simulink model "v2021_10_27_Modello_SITL_AENEA_2020b"  (R2020b)
settings: Solver=ode4  StartTime=0.0  StopTime=150  FixedStep=0.01  RelTol=1e-3
values from neighbouring files (symbols this model uses):
  alphavec_rad = [-0.10471975512 -0.0872664625997 -0.0698131700798 -0.0523598775598 -0.0349065850399 -0.0174532925199 0 0.0174532925199 0.0349065850399 0.0523598775598 0.0698131700798 0.0872664625997 ... (13 elements, 1x13)]    [datiAerodinamiciAENEA.mat]    (also in v2021_10_27_calcoloAerodinamica.m = deg2rad(alphavec))
  attuatore_Amax = 20*(pi/180)    (= 0.349065850399)    [v2021_10_27_avvioSITL.m]    (also in v2021_10_27_calcoloAerodinamica.m)
  attuatore_Emax = 25*(pi/180)    (= 0.436332312999)    [v2021_10_27_avvioSITL.m]    (also in v2021_10_27_calcoloAerodinamica.m)
  attuatore_Rmax = 25*(pi/180)    (= 0.436332312999)    [v2021_10_27_avvioSITL.m]    (also in v2021_10_27_calcoloAerodinamica.m)
  b = 2.62    [datiAerodinamiciAENEA.mat]    (also in derivateROSKAM_new.m; v2021_10_27_calcoloAerodinamica.m)
  beta_phi = 1/10.5600    (= 0.094696969697)    [Load_modello_sensori.m]
  beta_psi = 1/170    (= 0.00588235294118)    [Load_modello_sensori.m]
  beta_theta = 1/10.5000    (= 0.0952380952381)    [Load_modello_sensori.m]
  betavec_rad = [-0.209439510239 -0.13962634016 -0.0698131700798 0 0.0698131700798 0.13962634016 0.209439510239]    [datiAerodinamiciAENEA.mat]    (also in v2021_10_27_calcoloAerodinamica.m = deg2rad(betavec))
  c = 0.32    [datiAerodinamiciAENEA.mat]    (also in derivateROSKAM_new.m; v2021_10_27_calcoloAerodinamica.m)
  cbar = 0.32    [datiAerodinamiciAENEA.mat]    (also in v2021_10_27_calcoloAerodinamica.m)
  CD0 = 0.2    [datiAerodinamiciAENEA.mat]    (also in v2021_10_27_calcoloAerodinamica.m = 0.024)
  CldA = KCldA(1)*180/pi    [Alettoni.m]    (also in datiAerodinamiciAENEA.mat = 0.490103315517)
  CLdE = KCLdE(1)*180/pi    [Equilibratore.m]    (also in datiAerodinamiciAENEA.mat = 0.809101149087)
  CldR = 0.0568697125654    [datiAerodinamiciAENEA.mat]
  Clp = -0.4318    [datiAerodinamiciAENEA.mat]    (also in derivateROSKAM_new.m = clp_w+2*(Zv/b)^2*cy_betav+Clp_tail; v2021_10_27_calcoloAerodinamica.m)
  CLq = 8.13    [datiAerodinamiciAENEA.mat]    (also in v2021_10_27_calcoloAerodinamica.m)
  Clr = 0.1459    [datiAerodinamiciAENEA.mat]    (also in derivateROSKAM_new.m = cl*clr_cl-(2/b^2)*(lv*cos(alpha)+Zv*sin(alpha))*(Zv*cos(alph; v2021_10_27_calcoloAerodinamica.m)
  CmdE = KCmdE(1)*180/pi    [Equilibratore.m]    (also in datiAerodinamiciAENEA.mat = -3.59730623976)
  Cmq = -23.24    [datiAerodinamiciAENEA.mat]    (also in derivateROSKAM_new.m = -K*cL_alphaw*((AR*(2*(Xw/c)^2+0.5*(Xw/c))/(AR+2))+1/8)-2*cL_; v2021_10_27_calcoloAerodinamica.m)
  CndA = KCndA(1)*180/pi    [Alettoni.m]    (also in datiAerodinamiciAENEA.mat = -0.0456969018066)
  CndR = -0.162544523826    [datiAerodinamiciAENEA.mat]
  Cnp = 0.000294    [datiAerodinamiciAENEA.mat]    (also in derivateROSKAM_new.m = -clp_w*tan(alpha)+Clp*tan(alpha)-(2/b)*(lv*cos(alpha)+Zv*sin; v2021_10_27_calcoloAerodinamica.m = 0.007507)
  Cnr = -0.4872    [datiAerodinamiciAENEA.mat]    (also in derivateROSKAM_new.m = (Cnr_Clquadro)*cl^2+(cnr_cd0)*cd0+(2/b^2)*(lv*cos(alpha)+Zv*; v2021_10_27_calcoloAerodinamica.m)
  CYdA = KCYdA(1)*180/pi    [Alettoni.m]    (also in datiAerodinamiciAENEA.mat = -0.0146577407549)
  CYdR = -0.298131751664    [datiAerodinamiciAENEA.mat]
  CYp = 0.050728    [datiAerodinamiciAENEA.mat]    (also in v2021_10_27_calcoloAerodinamica.m)
  CYr = 0.358925    [datiAerodinamiciAENEA.mat]    (also in v2021_10_27_calcoloAerodinamica.m)
  delay_ahrs = 0    [Load_modello_sensori.m]
  delay_bmp = 0    [Load_modello_sensori.m]
  delay_gps = 0    [Load_modello_sensori.m]
  deltaAtrim = 0    [v2021_10_27_avvioSITL.m]
  deltaEtrim = (Cm0*CL_alpharad+Cm_alpharad*CLtrim)/(CL_alpharad*CmdE)    [calcoloDatiIniziali.m]    (also in v2021_10_27_avvioSITL.m = 0)
  deltaRtrim = 0    [v2021_10_27_avvioSITL.m]
  deltaTtrim = 0.1    [v2021_10_27_avvioSITL.m]
  Dprop = 0.5334    [datiAerodinamiciAENEA.mat]    (also in v2021_10_27_calcoloAerodinamica.m)
  g = [0 0 9.81]    [datiAerodinamiciAENEA.mat]    (also in v2021_10_27_calcoloAerodinamica.m = [0 0 9.81]')
  HINI = -State0.Pos0(3)    [v2021_10_27_avvioSITL.m]
  J_vec = [0 0.03 0.06 0.09 0.11 0.14 0.17 0.2 0.23 0.26 0.28 0.31 ... (30 elements, 30x1)]    [datiAerodinamiciAENEA.mat]
  Jeng = 0    [datiAerodinamiciAENEA.mat]    (also in v2021_10_27_calcoloAerodinamica.m)
  Jprop = 0.00422031414    [datiAerodinamiciAENEA.mat]    (also in v2021_10_27_calcoloAerodinamica.m)
  latitudineINI = 41.88754294247101*pi/180    (= 0.731075539917)    [v2021_10_27_avvioSITL.m]
  longitudineINI = 12.539364533818434*pi/180    (= 0.218853197223)    [v2021_10_27_avvioSITL.m]
  mean_ax = 0*0.0392    (= 0)    [Load_modello_sensori.m]
  mean_ay = -0*0.0598    (= 0)    [Load_modello_sensori.m]
  mean_az = 0*0.0384    (= 0)    [Load_modello_sensori.m]
  mean_p = 0*1.5184e-06    (= 0)    [Load_modello_sensori.m]
  mean_q = 0*2.9671e-05    (= 0)    [Load_modello_sensori.m]
  mean_r = 0*5.4105e-05    (= 0)    [Load_modello_sensori.m]
  P_ref = 1.0074e+05    (= 100740)    [Load_modello_sensori.m]
  PWM_Aileron = rad2deg(deltaAtrim)*9+1503    [v2021_10_27_avvioSITL.m]
  PWM_Elevator = rad2deg(deltaEtrim)*(447/50)+(3007/2)    [v2021_10_27_avvioSITL.m]
  PWM_Rudder = rad2deg(deltaRtrim)*(447/50)+(3007/2)    [v2021_10_27_avvioSITL.m]
  PWM_Throttle = (deltaTtrim)*800+1100    (= 1180)    [v2021_10_27_avvioSITL.m]
  q = prediction(11)    [f_pred_F1B.m]
  r = prediction(12)    [f_pred_F1B.m]
  rACtG = [-1.334 0 -0.2103]    [datiAerodinamiciAENEA.mat]    (also in v2021_10_27_calcoloAerodinamica.m = rACtP-rGP)
  rACwG = [-0.0589 0 -0.1645]    [datiAerodinamiciAENEA.mat]    (also in v2021_10_27_calcoloAerodinamica.m = rACwP-rGP)
  rAHRSG = [0 0 0.1075]    [datiAerodinamiciAENEA.mat]    (also in v2021_10_27_calcoloAerodinamica.m = rAHRSP-rGP)
  rho = 1.2133    [datiAerodinamiciAENEA.mat]    (also in derivateROSKAM_new.m = 1.16123787958; v2021_10_27_calcoloAerodinamica.m)
  rLEG = [0.0211 0 -0.1645]    [datiAerodinamiciAENEA.mat]    (also in v2021_10_27_calcoloAerodinamica.m = rLEP-rGP)
  rmglG = [-0.2319 -0.2 0.3925]    [datiAerodinamiciAENEA.mat]    (also in v2021_10_27_calcoloAerodinamica.m = rmglP-rGP)
  rmgrG = [-0.2319 0.2 0.3925]    [datiAerodinamiciAENEA.mat]    (also in v2021_10_27_calcoloAerodinamica.m = rmgrP-rGP)
  rngG = [0.2969 0 0.3925]    [datiAerodinamiciAENEA.mat]    (also in v2021_10_27_calcoloAerodinamica.m = rngP-rGP)
  rNPG = [-0.2442 0 -0.1645]    [datiAerodinamiciAENEA.mat]    (also in v2021_10_27_calcoloAerodinamica.m = rNPP-rGP)
  rPG = [0.5 0 -0.1075]    [datiAerodinamiciAENEA.mat]    (also in v2021_10_27_calcoloAerodinamica.m = -rGP)
  Rprop = 0.2667    [datiAerodinamiciAENEA.mat]    (also in v2021_10_27_calcoloAerodinamica.m)
  S = 0.8384    [datiAerodinamiciAENEA.mat]    (also in derivateROSKAM_new.m; v2021_10_27_calcoloAerodinamica.m)
  seed_ahrs = randi([0 2000],1,1)    [Load_modello_sensori.m]
  seed_baro = randi([0 2000],1,1)    [Load_modello_sensori.m]
  seed_gps = randi([0 2000],1,1)    [Load_modello_sensori.m]
  sensori_FreqCampionamento_pitot = 0.02    [v2021_10_27_avvioSITL.m]
  sensori_RumoreSampleTime = 0.02    [v2021_10_27_avvioSITL.m]
  sensori_varianza = 0.0000    (= 0)    [v2021_10_27_avvioSITL.m]
  Std_con_lat = 2.7349e-07    [Load_modello_sensori.m]
  Std_con_long = 1.3733e-06    [Load_modello_sensori.m]
  Std_vel = 0.05    [Load_modello_sensori.m]
  T0_ref = 25    [Load_modello_sensori.m]
  Ta_lat = 10^2    (= 100)    [Load_modello_sensori.m]
  Ta_long = 10^2    (= 100)    [Load_modello_sensori.m]
  Ts_ahrs = 0.02    [Load_modello_sensori.m]
  Ts_bmp = 0.02    [Load_modello_sensori.m]
  Ts_gps = 0.2    [Load_modello_sensori.m]
  tsamp = 0.02    [v2021_10_27_avvioSITL.m]
  V_cruise = input('inserire un valore desiderato per V_cruise: ')    [trimCalc.m]
  Var_heading_static = 0.1    [Load_modello_sensori.m]
  Var_V_hor_static = 0.25    [Load_modello_sensori.m]
  W = [0 0 92.214]    [datiAerodinamiciAENEA.mat]    (also in derivateROSKAM_new.m = 112.815; v2021_10_27_calcoloAerodinamica.m = m*g)
  White_ax = 1.486e-04    (= 0.0001486)    [Load_modello_sensori.m]
  White_ay = 9.403e-05    [Load_modello_sensori.m]
  White_az = 1.648e-04    (= 0.0001648)    [Load_modello_sensori.m]
  White_gm_phi = 3.2740e-05    (= 3.274e-05)    [Load_modello_sensori.m]
  White_gm_psi = 2.9162e-04    (= 0.00029162)    [Load_modello_sensori.m]
  White_gm_theta = 2.4704e-05    [Load_modello_sensori.m]
  White_p = 2.934e-05    [Load_modello_sensori.m]
  White_pressione = 10.18    [Load_modello_sensori.m]
  White_r = 3.258e-05    [Load_modello_sensori.m]
  WP_AL = [     0 20 0 0 41.807822 12.589274 3 ... (first row only)    [v2021_10_27_avvioSITL.m]
  WP_db_info = [0 0 0 0 1 3;              0 0 0 0 2 3;              0 0 0 0 3 3;              0 0 0 0 0 0]    [v2021_10_27_avvioSITL.m]
  WP_db_param = [              0 0 17 0 41.887798530888304, 12.537905412104232 75;              0 0 20 0 41.89052329007801, 12.492437426923948 65;              0 0 24 0 41.93506891472633, 12.504514543566634 80;              0 0 0 0 0 0 0 ... (first row only)    [v2021_10_27_avvioSITL.m]
  Zeng = -0.1075    [datiAerodinamiciAENEA.mat]    (also in v2021_10_27_calcoloAerodinamica.m = rPG(3))
  Zpista = 0    [v2021_10_27_avvioSITL.m]
undefined symbols (not defined in the file or in its folder): Earth, F, h_home, matricepolinomi, MIL, Receive, Send, State0, WGS84
libraries: simulink_extras x27, aerolibfltsims x5, aerolibwind2 x3, aerolibasang x2, simulink x2, shared6dof x1, pid_lib x1, aerolibatmos2 x1, aerolibanimutils x1
(part 3 of 3)

== system v2021_10_27_Modello_SITL_AENEA_2020b/AENEA /AENEA II_SITL1/Weight ==
  LBE : Inport
  Vect_Costanti : Inport  Port=2
  Bus Selector : BusSelector  OutputSignals=Coef_Geometrici.W
  Display1 : Display
  Display3 : Display
  Product3 : Product  Multiplication=Matrix(*)
  "Forzapeso " : Outport  VectorParamsAs1DForOutWhenUnconnected=off
  wires:
  Product3/1 -> "Forzapeso "/1, Display3/1
  LBE/1 -> Product3/1
  Vect_Costanti/1 -> Bus Selector/1
  Bus Selector/1 -> Display1/1, Product3/2  "<W>"

== system v2021_10_27_Modello_SITL_AENEA_2020b/AENEA /toSensors/Calc_GS ==
  In1 : Inport
  Add : Sum
  Demux : Demux  Outputs=3
  Sqrt : Sqrt  SaturateOnIntegerOverflow=on
  Square1 : Math  Operator=square  SignedPower=on  SaturateOnIntegerOverflow=on
  Square2 : Math  Operator=square  SignedPower=on  SaturateOnIntegerOverflow=on
  Terminator : Terminator
  GS : Outport  VectorParamsAs1DForOutWhenUnconnected=off
  wires:
  In1/1 -> Demux/1
  Demux/2 -> Square1/1
  Demux/1 -> Square2/1
  Demux/3 -> Terminator/1
  Square2/1 -> Add/1
  Square1/1 -> Add/2
  Add/1 -> Sqrt/1
  Sqrt/1 -> GS/1

== system v2021_10_27_Modello_SITL_AENEA_2020b/AENEA /toSensors/Calc_heading ==
  In1 : Inport
  Atan2 : Trigonometry  Operator=atan2
  Demux : Demux  Outputs=3
  Terminator : Terminator
  Heading : Outport  VectorParamsAs1DForOutWhenUnconnected=off
  wires:
  In1/1 -> Demux/1
  Demux/3 -> Terminator/1
  Demux/2 -> Atan2/1
  Demux/1 -> Atan2/2
  Atan2/1 -> Heading/1

== system v2021_10_27_Modello_SITL_AENEA_2020b/AENEA /toSensors/To_Lat_Long_MSL ==
  note: Navigation equation
  note: Position derivatives
  V_NED : Inport
  Demux1 : Demux  Outputs=3
      settings: DisplayOption=none
  Demux3 : Demux  Outputs=3
      settings: DisplayOption=none
  Gain : Gain  Gain=-1
  Latitude Bound : Subsystem  mask(Latitude bound){}
      mask help: Bounds the latitude to [-pi/2, pi/2]. When the lower bound is exceeded the latitude is increasing again; when the upper bound is exceeded the latitude is decreasing.
  Longitude Bound : Subsystem  mask(Longitude bound){}
      mask help: Bounds the longitude to [-pi, pi]. When -pi bound is exceeded the longitude wraps back to pi; when the pi bound is exceeded the longitude wraps back to -pi.
  Mux : Mux  Inputs=3
  Mux1 : Mux  Inputs=3
  Position Integrator2 : Integrator  InitialCondition=[latitudineINI longitudineINI HINI]
  Radius at Geocentric Latitude : aerolibasang/Radius at Geocentric Latitude  units=Metric (MKS)  ptype=Earth (WGS84)  F=1/298.257223563  R=6378137
      settings: SourceProductBaseCode=AE
  Sum : Sum  Inputs=|++  InputSameDT=on  SaturateOnIntegerOverflow=on  OutDataTypeStr=Inherit: Same as first input
  Sum1 : Sum  Inputs=|++  InputSameDT=on  SaturateOnIntegerOverflow=on  OutDataTypeStr=Inherit: Same as first input
  Ve/(Rn+h)cos(phi) : Product  Inputs=*//  InputSameDT=on  SaturateOnIntegerOverflow=on  OutDataTypeStr=Inherit: Same as first input
  Vn/(Rm+h) : Product  Inputs=*/  InputSameDT=on  SaturateOnIntegerOverflow=on  OutDataTypeStr=Inherit: Same as first input
  cos(phi) : Trigonometry  Operator=cos
  Position : Outport  VectorParamsAs1DForOutWhenUnconnected=off
  wires:
  Latitude Bound/1(Out) -> cos(phi)/1, Radius at Geocentric Latitude/1, Mux1/1  "lat_optim"
  Longitude Bound/1(Out) -> Mux1/2
  cos(phi)/1 -> Ve/(Rn+h)cos(phi)/3
  Sum1/1 -> Ve/(Rn+h)cos(phi)/2
  Demux3/1 -> Latitude Bound/1(In)
  Ve/(Rn+h)cos(phi)/1 -> Mux/2
  Demux3/2 -> Longitude Bound/1(In)
  Mux1/1 -> Position/1
  Position Integrator2/1 -> Demux3/1
  Demux1/2 -> Ve/(Rn+h)cos(phi)/1
  Mux/1 -> Position Integrator2/1
  Sum/1 -> Vn/(Rm+h)/2
  V_NED/1 -> Demux1/1
  Vn/(Rm+h)/1 -> Mux/1
  Demux3/3 -> Sum/2, Sum1/2, Mux1/3
  Demux1/1 -> Vn/(Rm+h)/1
  Gain/1 -> Mux/3
  Demux1/3 -> Gain/1
  Radius at Geocentric Latitude/1 -> Sum1/1, Sum/1

== system v2021_10_27_Modello_SITL_AENEA_2020b/Ricezione segnali2/Subsystem1/AILERON ==
  In1 : Inport
  Constant : Constant  Value=167
  Gain : Gain  Gain=1/9
  Sum : Sum  Inputs=|+-
  Out1 : Outport  VectorParamsAs1DForOutWhenUnconnected=off
  wires:
  Gain/1 -> Sum/1
  Constant/1 -> Sum/2
  Sum/1 -> Out1/1
  In1/1 -> Gain/1

== system v2021_10_27_Modello_SITL_AENEA_2020b/Ricezione segnali2/Subsystem1/ELEVATOR ==
  In1 : Inport
  Constant : Constant  Value=75175/447
  Gain : Gain  Gain=50/447
  Sum : Sum  Inputs=|+-
  Out1 : Outport  VectorParamsAs1DForOutWhenUnconnected=off
  wires:
  In1/1 -> Gain/1
  Constant/1 -> Sum/2
  Sum/1 -> Out1/1
  Gain/1 -> Sum/1

== system v2021_10_27_Modello_SITL_AENEA_2020b/Ricezione segnali2/Subsystem1/RUDDER ==
  In1 : Inport
  Constant : Constant  Value=75175/447
  Gain : Gain  Gain=50/447
  Sum : Sum  Inputs=|+-
  Out1 : Outport  VectorParamsAs1DForOutWhenUnconnected=off
  wires:
  Gain/1 -> Sum/1
  Constant/1 -> Sum/2
  Sum/1 -> Out1/1
  In1/1 -> Gain/1

== system v2021_10_27_Modello_SITL_AENEA_2020b/Ricezione segnali2/Subsystem1/THROTTLE ==
  In1 : Inport
  Constant : Constant  Value=11/8
  Constant2 : Constant  Value=0
  Gain : Gain  Gain=1/800
  Sum : Sum  Inputs=|+-
  Switch : Switch  Criteria=u2 > Threshold  Threshold=0.003
  Out1 : Outport  VectorParamsAs1DForOutWhenUnconnected=off
  wires:
  In1/1 -> Gain/1
  Constant/1 -> Sum/2
  Gain/1 -> Sum/1
  Switch/1 -> Out1/1
  Sum/1 -> Switch/1, Switch/2
  Constant2/1 -> Switch/3

== system v2021_10_27_Modello_SITL_AENEA_2020b/AENEA /AENEA II_SITL1/Forze aerodinamiche/Forze assi vento//q ==
  Vect_Comandi : Inport
  Vect_Costanti : Inport  Port=2
  "Vbpolare " : Inport  Port=3
  ωb : Inport  Port=4
  Bus Creator : BusCreator  Inputs=3
  Bus Selector : BusSelector  OutputSignals=deltaE
  Bus Selector1 : BusSelector  OutputSignals=p,r,q
  Display : Display
  Gain4 : Gain  Gain=-1
  Gain5 : Gain  Gain=-1
  Scope : Scope
  Subsystem : Subsystem
  Subsystem1 : Subsystem
  Subsystem2 : Subsystem
  FA_W/q : Outport  VectorParamsAs1DForOutWhenUnconnected=off
  CL : Outport  Port=2  VectorParamsAs1DForOutWhenUnconnected=off
  wires:
  Bus Selector/1 -> Subsystem2/2(deltaE)  "<deltaE>"
  Subsystem/1(CD) -> Display/1, Scope/1, Gain4/1
  Subsystem2/1(CL) -> CL/1, Gain5/1
  Vect_Costanti/1 -> Subsystem2/3(Vect_Costanti), Subsystem1/3(Vect_Costanti), Subsystem/1(Vect_Costanti)
  Vect_Comandi/1 -> Subsystem1/4(Vect_Comandi), Bus Selector/1
  "Vbpolare "/1 -> Subsystem1/5("Vbpolare "), Subsystem2/4("Vbpolare "), Subsystem/2("Vbpolare ")
  ωb/1 -> Bus Selector1/1
  Bus Selector1/1 -> Subsystem1/1(p)  "<p>"
  Bus Selector1/3 -> Subsystem2/1(q)  "<q>"
  Bus Selector1/2 -> Subsystem1/2(r)  "<r>"
  Bus Creator/1 -> FA_W/q/1
  Gain5/1 -> Bus Creator/3  "CL"
  Subsystem1/1("CY ") -> Bus Creator/2  "CY"
  Gain4/1 -> Bus Creator/1  "CD"

== system v2021_10_27_Modello_SITL_AENEA_2020b/AENEA /AENEA II_SITL1/Forze aerodinamiche/Momenti //press din ==
  Vect_Comandi : Inport
  Vect_Costanti : Inport  Port=2
  "Vbpolare " : Inport  Port=3
  ωb : Inport  Port=4
  Bus Creator : BusCreator  Inputs=3
  Bus Selector : BusSelector  OutputSignals=Coef_Geometrici.S*b,Coef_Geometrici.S*cbar
  Product : Product
  Product1 : Product
  Product3 : Product
  Subsystem3 : Subsystem
  Subsystem4 : Subsystem
  Subsystem5 : Subsystem
  MA_B/q : Outport  VectorParamsAs1DForOutWhenUnconnected=off
  wires:
  Subsystem5/1(Cn) -> Product3/2
  Subsystem4/1(Cm) -> Product1/2
  Subsystem3/1(Cl) -> Product/2
  Vect_Costanti/1 -> Bus Selector/1, Subsystem3/1(Vect_Costanti), Subsystem5/1(Vect_Costanti), Subsystem4/1(Vect_Costanti)
  Vect_Comandi/1 -> Subsystem4/2(Vect_Comandi), Subsystem3/2(Vect_Comandi), Subsystem5/2(Vect_Comandi)
  "Vbpolare "/1 -> Subsystem5/3("Vbpolare "), Subsystem4/3("Vbpolare "), Subsystem3/3("Vbpolare ")
  ωb/1 -> Subsystem5/4(ωb), Subsystem4/4(ωb), Subsystem3/4(ωb)
  Bus Selector/1 -> Product3/1, Product/1  "<S*b>"
  Bus Selector/2 -> Product1/1  "<S*cbar>"
  Bus Creator/1 -> MA_B/q/1
  Product/1 -> Bus Creator/1  "Cl"
  Product1/1 -> Bus Creator/2  "Cm"
  Product3/1 -> Bus Creator/3  "Cn"

== system v2021_10_27_Modello_SITL_AENEA_2020b/AENEA /AENEA II_SITL1/Propulsione1/LUT ELICA  ==
  J : Inport
  RPM : Inport  Port=2
  Constant : Constant  Value=matricepolinomi  VectorParams1D=off
  MATLAB Function : MATLAB Function  TreatAsAtomicUnit=on
  Ct : Outport  VectorParamsAs1DForOutWhenUnconnected=off
  Cp : Outport  Port=2  VectorParamsAs1DForOutWhenUnconnected=off
  wires:
  MATLAB Function/2(Cp) -> Cp/1  "Cp"
  J/1 -> MATLAB Function/1(J)
  Constant/1 -> MATLAB Function/3(matricepolinomi)
  MATLAB Function/1(Ct) -> Ct/1  "Ct"
  RPM/1 -> MATLAB Function/2(RPM)

== system v2021_10_27_Modello_SITL_AENEA_2020b/AENEA /AENEA II_SITL1/Propulsione1/LUT ELICA 1 ==
  J : Inport
  RPM : Inport  Port=2
  2-D Lookup Table : Lookup_n-D  BreakpointsForDimension1=J_vec  BreakpointsForDimension2=RPM_vec(2:end)  Table=Ct(2:end,2:end)  InternalRulePriority=Speed  RndMeth=Simplest  InputSameDT=on
      settings: InputPortMap=u0,u1
  2-D Lookup Table1 : Lookup_n-D  BreakpointsForDimension1=J_vec  BreakpointsForDimension2=RPM_vec(2:end)  Table=Cp(2:end,2:end)  InternalRulePriority=Speed  RndMeth=Simplest  InputSameDT=on
      settings: InputPortMap=u0,u1
  Ct : Outport  VectorParamsAs1DForOutWhenUnconnected=off
  Cp : Outport  Port=2  VectorParamsAs1DForOutWhenUnconnected=off
  wires:
  RPM/1 -> 2-D Lookup Table/2, 2-D Lookup Table1/2
  J/1 -> 2-D Lookup Table1/1, 2-D Lookup Table/1
  2-D Lookup Table1/1 -> Cp/1
  2-D Lookup Table/1 -> Ct/1

== system v2021_10_27_Modello_SITL_AENEA_2020b/AENEA /AENEA II_SITL1/Propulsione1/Subsystem1 ==
  T : Inport
  P : Inport  Port=2
  RPS : Inport  Port=3
  V_cost : Inport  Port=4
  Bus Selector : BusSelector  OutputSignals=Coef_Propulsivi.Zeng
  Constant : Constant  Value=0
  Constant1 : Constant  Value=0
  Divide : Product  Inputs=*/
  Divide1 : Product  Inputs=**
  Gain : Gain  Gain=2*pi
  Gain1 : Gain  Gain=-1
  Mux : Mux  Inputs=3
  Mux1 : Mux  Inputs=3
  Fthrust : Outport  VectorParamsAs1DForOutWhenUnconnected=off
  "Mthrust " : Outport  Port=2  VectorParamsAs1DForOutWhenUnconnected=off
  wires:
  T/1 -> Divide1/2, Mux/1
  Constant/1 -> Mux/2, Mux/3
  Mux/1 -> Fthrust/1
  RPS/1 -> Gain/1
  P/1 -> Divide/1
  Gain/1 -> Divide/2
  Gain1/1 -> Mux1/1
  Divide/1 -> Gain1/1
  Divide1/1 -> Mux1/2
  Constant1/1 -> Mux1/3
  Mux1/1 -> "Mthrust "/1
  V_cost/1 -> Bus Selector/1
  Bus Selector/1 -> Divide1/1  "<Zeng>"

== system v2021_10_27_Modello_SITL_AENEA_2020b/AENEA /AENEA II_SITL1/Propulsione1/Subsystem2 ==
  T : Inport
  P : Inport  Port=2
  RPS : Inport  Port=3
  Constant : Constant  Value=0
  Constant1 : Constant  Value=0
  Divide : Product  Inputs=*/
  Gain : Gain  Gain=2*pi
  Gain1 : Gain  Gain=-1
  Mux : Mux  Inputs=3
  Mux1 : Mux  Inputs=3
  "xprop " : Gain  Gain=-0.15
  Fthrust : Outport  VectorParamsAs1DForOutWhenUnconnected=off
  "Mthrust " : Outport  Port=2  VectorParamsAs1DForOutWhenUnconnected=off
  wires:
  T/1 -> "xprop "/1, Mux/1
  Constant/1 -> Mux/2, Mux/3
  Mux/1 -> Fthrust/1
  RPS/1 -> Gain/1
  P/1 -> Divide/1
  Gain/1 -> Divide/2
  Gain1/1 -> Mux1/1
  Divide/1 -> Gain1/1
  "xprop "/1 -> Mux1/2
  Constant1/1 -> Mux1/3
  Mux1/1 -> "Mthrust "/1

== system v2021_10_27_Modello_SITL_AENEA_2020b/AENEA /toSensors/To_Lat_Long_MSL/Latitude Bound ==
  In : Inport
  2pi : Constant  Value=2*pi
  ChSign : Gain  Gain=-1  SaturateOnIntegerOverflow=on  OutDataTypeStr=Inherit: Same as input  ParamDataTypeStr=Inherit: Same as input
  Math Function : Math  Operator=mod  SignedPower=on  SaturateOnIntegerOverflow=on
  Math Function1 : Math  Operator=mod  SignedPower=on  SaturateOnIntegerOverflow=on
  Sum1 : Sum  Inputs=|+-  InputSameDT=on  SaturateOnIntegerOverflow=on  OutDataTypeStr=Inherit: Same as first input
  Sum2 : Sum  Inputs=|++  InputSameDT=on  SaturateOnIntegerOverflow=on  OutDataTypeStr=Inherit: Same as first input
  Switch : Switch  Threshold=pi  SaturateOnIntegerOverflow=on  InputSameDT=on
  pi : Constant  Value=pi
  pi/2 : Constant  Value=pi/2
  Out : Outport  VectorParamsAs1DForOutWhenUnconnected=off
  wires:
  pi/1 -> Math Function/2
  Math Function/1 -> Sum1/1
  pi/2/1 -> Sum1/2, Sum2/2
  Sum1/1 -> ChSign/1, Switch/3
  Math Function1/1 -> Switch/2
  Switch/1 -> Out/1
  In/1 -> Sum2/1
  Sum2/1 -> Math Function/1, Math Function1/1
  ChSign/1 -> Switch/1
  2pi/1 -> Math Function1/2

== system v2021_10_27_Modello_SITL_AENEA_2020b/AENEA /toSensors/To_Lat_Long_MSL/Longitude Bound ==
  In : Inport
  2pi : Constant  Value=2*pi
  Math Function : Math  Operator=mod  SignedPower=on  SaturateOnIntegerOverflow=on
  Sum1 : Sum  Inputs=|+-  InputSameDT=on  SaturateOnIntegerOverflow=on  OutDataTypeStr=Inherit: Same as first input
  Sum2 : Sum  Inputs=|++  InputSameDT=on  SaturateOnIntegerOverflow=on  OutDataTypeStr=Inherit: Same as first input
  pi : Constant  Value=pi
  Out : Outport  VectorParamsAs1DForOutWhenUnconnected=off
  wires:
  Sum1/1 -> Out/1
  pi/1 -> Sum1/2, Sum2/2
  Sum2/1 -> Math Function/1
  In/1 -> Sum2/1
  2pi/1 -> Math Function/2
  Math Function/1 -> Sum1/1

== system v2021_10_27_Modello_SITL_AENEA_2020b/AENEA /AENEA II_SITL1/Forze aerodinamiche/Forze assi vento//q/Subsystem ==
  note: CD=CD(alpha_x,beta)
  Vect_Costanti : Inport
  "Vbpolare " : Inport  Port=2
  2-D Lookup Table : Lookup_n-D  BreakpointsForDimension1=alphavec_rad  BreakpointsForDimension2=betavec_rad  Table=CD(2:end,2:end)  InternalRulePriority=Speed  RndMeth=Simplest  InputSameDT=on
      settings: InputPortMap=u0,u1
  Bus Selector : BusSelector  OutputSignals=Coef_Aerodinamici.Coef_Forze.CD0
  Bus Selector1 : BusSelector  OutputSignals=α,β
  Sum1 : Sum  Inputs=|++
  CD : Outport  VectorParamsAs1DForOutWhenUnconnected=off
  wires:
  2-D Lookup Table/1 -> Sum1/1
  Sum1/1 -> CD/1
  Bus Selector/1 -> Sum1/2  "<CD0>"
  Vect_Costanti/1 -> Bus Selector/1
  Bus Selector1/1 -> 2-D Lookup Table/1  "<α>"
  "Vbpolare "/1 -> Bus Selector1/1
  Bus Selector1/2 -> 2-D Lookup Table/2  "<β>"

== system v2021_10_27_Modello_SITL_AENEA_2020b/AENEA /AENEA II_SITL1/Forze aerodinamiche/Forze assi vento//q/Subsystem1 ==
  note: CY=CY(alpha_x,beta)+CY_p*p+CY_r*r+CY_deltaA*deltaA+CY_deltaR*deltaR
  p : Inport
  r : Inport  Port=2
  Vect_Costanti : Inport  Port=3
  Vect_Comandi : Inport  Port=4
  "Vbpolare " : Inport  Port=5
  2-D Lookup Table : Lookup_n-D  BreakpointsForDimension1=alphavec_rad  BreakpointsForDimension2=betavec_rad  Table=CY(2:end,2:end)  InternalRulePriority=Speed  RndMeth=Simplest  InputSameDT=on
      settings: InputPortMap=u0,u1
  Bus Selector : BusSelector  OutputSignals=deltaR,deltaA
  Bus Selector1 : BusSelector  OutputSignals=Coef_Geometrici.b/2,Coef_Aerodinamici.Coef_Forze.CYp,Coef_Aerodinamici.Coef_Forze.CYr,Coef_Aerodinamici.Coef_Forze.CYdR,Coef_Aerodinamici.Coef_Forze.CYdA
  Bus Selector2 : BusSelector  OutputSignals=α,β,V
  Mux : Mux
  Mux1 : Mux
  Product : Product
  Product3 : Product
  Saturation : Saturate  UpperLimit=0.1  LowerLimit=-0.1
  Sum : Sum  Inputs=5
  "controllo divisione per zero Yp " : MATLAB Function  TreatAsAtomicUnit=on
  controllo divisione per zero Yr : MATLAB Function  TreatAsAtomicUnit=on
  "CY " : Outport  VectorParamsAs1DForOutWhenUnconnected=off
  wires:
  Bus Selector1/2 -> Mux/1  "<CYp>"
  p/1 -> Mux/2
  "controllo divisione per zero Yp "/1(y) -> Sum/2
  Sum/1 -> "CY "/1
  r/1 -> Mux1/1
  2-D Lookup Table/1 -> Saturation/1
  Bus Selector1/4 -> Product/1  "<CYdR>"
  Bus Selector/1 -> Product/2  "<deltaR>"
  Bus Selector1/5 -> Product3/1  "<CYdA>"
  Bus Selector/2 -> Product3/2  "<deltaA>"
  Product/1 -> Sum/4
  Product3/1 -> Sum/5
  Vect_Comandi/1 -> Bus Selector/1
  Vect_Costanti/1 -> Bus Selector1/1
  Bus Selector1/3 -> Mux1/3  "<CYr>"
  Bus Selector1/1 -> Mux/3, Mux1/2  "<b/2>"
  Bus Selector2/1 -> 2-D Lookup Table/1  "<α>"
  "Vbpolare "/1 -> Bus Selector2/1
  Bus Selector2/3 -> Mux/4, Mux1/4  "<V>"
  Bus Selector2/2 -> 2-D Lookup Table/2  "<β>"
  Mux/1 -> "controllo divisione per zero Yp "/1(u)
  Mux1/1 -> controllo divisione per zero Yr/1(u)
  controllo divisione per zero Yr/1(y) -> Sum/3
  Saturation/1 -> Sum/1

== system v2021_10_27_Modello_SITL_AENEA_2020b/AENEA /AENEA II_SITL1/Forze aerodinamiche/Forze assi vento//q/Subsystem2 ==
  note: CL=CL(ALPHA_X,BETA)+CL_q*q+CL_de*de
  q : Inport
  deltaE : Inport  Port=2
  Vect_Costanti : Inport  Port=3
  "Vbpolare " : Inport  Port=4
  2-D Lookup Table : Lookup_n-D  BreakpointsForDimension1=alphavec_rad  BreakpointsForDimension2=betavec_rad  Table=CL(2:end,2:end)  InternalRulePriority=Speed  RndMeth=Simplest  InputSameDT=on
      settings: InputPortMap=u0,u1
  Bus Selector : BusSelector  OutputSignals=Coef_Aerodinamici.Coef_Forze.CLq,Coef_Aerodinamici.Coef_Forze.CLdE,Coef_Geometrici.cbar
  Bus Selector1 : BusSelector  OutputSignals=α,β,V
  Gain1 : Gain  Gain=2
  Mux : Mux
  Product4 : Product
  Sum : Sum  Inputs=3
  "controllo divisione per zero Lq " : MATLAB Function  TreatAsAtomicUnit=on
  CL : Outport  VectorParamsAs1DForOutWhenUnconnected=off
  wires:
  Sum/1 -> CL/1
  q/1 -> Mux/2
  Bus Selector/1 -> Mux/1  "<CLq>"
  Bus Selector/2 -> Product4/1  "<CLdE>"
  deltaE/1 -> Product4/2
  "controllo divisione per zero Lq "/1(y) -> Sum/2
  Product4/1 -> Sum/3
  2-D Lookup Table/1 -> Sum/1
  Vect_Costanti/1 -> Bus Selector/1
  Gain1/1 -> Mux/4
  Bus Selector/3 -> Mux/3  "<cbar>"
  Bus Selector1/1 -> 2-D Lookup Table/1  "<α>"
  "Vbpolare "/1 -> Bus Selector1/1
  Bus Selector1/3 -> Gain1/1  "<V>"
  Bus Selector1/2 -> 2-D Lookup Table/2  "<β>"
  Mux/1 -> "controllo divisione per zero Lq "/1(u)

== system v2021_10_27_Modello_SITL_AENEA_2020b/AENEA /AENEA II_SITL1/Forze aerodinamiche/Momenti //press din/Subsystem3 ==
  note: Gain aggiunto da CV e FM per modificare il CLBeta
  note: Cl=Cl(alpha_x,beta)+Cl_p*p+Cl_r*r+Cl_dA*dA+Cl_dR*dR
  Vect_Costanti : Inport
  Vect_Comandi : Inport  Port=2
  "Vbpolare " : Inport  Port=3
  ωb : Inport  Port=4
  2-D Lookup Table : Lookup_n-D  BreakpointsForDimension1=alphavec_rad  BreakpointsForDimension2=betavec_rad  Table=Cl(2:end,2:end)  InternalRulePriority=Speed  RndMeth=Simplest  InputSameDT=on
      settings: InputPortMap=u0,u1
  Bus Selector : BusSelector  OutputSignals=Coef_Aerodinamici.Coef_Momenti.Clp,Coef_Geometrici.b/2,Coef_Aerodinamici.Coef_Momenti.Clr,Coef_Aerodinamici.Coef_Momenti.CldA,Coef_Aerodinamici.Coef_Momenti.CldR
  Bus Selector1 : BusSelector  OutputSignals=deltaA,deltaR
  Bus Selector2 : BusSelector  OutputSignals=α,β,V
  Bus Selector3 : BusSelector  OutputSignals=p,r
  Gain4 : Gain  Gain=1.5
  Mux : Mux
  Mux1 : Mux
  Product2 : Product
  Product3 : Product
  Sum : Sum  Inputs=5
  "controllo divisione per zero lp " : MATLAB Function  TreatAsAtomicUnit=on
  "controllo divisione per zero lr " : MATLAB Function  TreatAsAtomicUnit=on
  Cl : Outport  VectorParamsAs1DForOutWhenUnconnected=off
  wires:
  Sum/1 -> Cl/1
  Bus Selector/3 -> Mux1/1  "<Clr>"
  Bus Selector1/2 -> Product3/2  "<deltaR>"
  Bus Selector1/1 -> Product2/2  "<deltaA>"
  Product3/1 -> Sum/5
  Product2/1 -> Sum/4
  "controllo divisione per zero lp "/1(y) -> Sum/2
  2-D Lookup Table/1 -> Gain4/1
  Gain4/1 -> Sum/1
  Vect_Costanti/1 -> Bus Selector/1
  Bus Selector/1 -> Mux/1  "<Clp>"
  Bus Selector/5 -> Product3/1  "<CldR>"
  Bus Selector/4 -> Product2/1  "<CldA>"
  Bus Selector/2 -> Mux1/2, Mux/3  "<b/2>"
  Vect_Comandi/1 -> Bus Selector1/1
  Bus Selector2/1 -> 2-D Lookup Table/1  "<α>"
  "Vbpolare "/1 -> Bus Selector2/1
  Bus Selector2/3 -> Mux1/4, Mux/4  "<V>"
  Bus Selector2/2 -> 2-D Lookup Table/2  "<β>"
  ωb/1 -> Bus Selector3/1
  Bus Selector3/1 -> Mux/2  "<p>"
  Bus Selector3/2 -> Mux1/3  "<r>"
  Mux/1 -> "controllo divisione per zero lp "/1(u)
  Mux1/1 -> "controllo divisione per zero lr "/1(u)
  "controllo divisione per zero lr "/1(y) -> Sum/3

== system v2021_10_27_Modello_SITL_AENEA_2020b/AENEA /AENEA II_SITL1/Forze aerodinamiche/Momenti //press din/Subsystem4 ==
  note: Cm=Cm(alpha_x,beta)+Cmq*q+Cm_deltaE*deltaE
  Vect_Costanti : Inport
  Vect_Comandi : Inport  Port=2
  "Vbpolare " : Inport  Port=3
  ωb : Inport  Port=4
  2-D Lookup Table : Lookup_n-D  BreakpointsForDimension1=alphavec_rad  BreakpointsForDimension2=betavec_rad  Table=Cm(2:end,2:end)  InternalRulePriority=Speed  RndMeth=Simplest  InputSameDT=on
      settings: InputPortMap=u0,u1
  Bus Selector : BusSelector  OutputSignals=deltaE
  Bus Selector1 : BusSelector  OutputSignals=Coef_Geometrici.cbar,Coef_Aerodinamici.Coef_Momenti.Cmq,Coef_Aerodinamici.Coef_Momenti.CmdE
  Bus Selector2 : BusSelector  OutputSignals=α,β,V
  Bus Selector3 : BusSelector  OutputSignals=q
  Gain1 : Gain  Gain=2
  Mux : Mux
  Product2 : Product
  Sum : Sum  Inputs=3
  "controllo divisione per zero mq " : MATLAB Function  TreatAsAtomicUnit=on
  Cm : Outport  VectorParamsAs1DForOutWhenUnconnected=off
  wires:
  Bus Selector1/2 -> Mux/1  "<Cmq>"
  Sum/1 -> Cm/1
  Gain1/1 -> Mux/4
  Bus Selector1/3 -> Product2/1  "<CmdE>"
  Bus Selector/1 -> Product2/2  "<deltaE>"
  Product2/1 -> Sum/3
  2-D Lookup Table/1 -> Sum/1
  Vect_Comandi/1 -> Bus Selector/1
  Vect_Costanti/1 -> Bus Selector1/1
  Bus Selector1/1 -> Mux/3  "<cbar>"
  Bus Selector2/3 -> Gain1/1  "<V>"
  "Vbpolare "/1 -> Bus Selector2/1
  Bus Selector2/1 -> 2-D Lookup Table/1  "<α>"
  Bus Selector2/2 -> 2-D Lookup Table/2  "<β>"
  ωb/1 -> Bus Selector3/1
  Bus Selector3/1 -> Mux/2  "<q>"
  Mux/1 -> "controllo divisione per zero mq "/1(u)
  "controllo divisione per zero mq "/1(y) -> Sum/2

== system v2021_10_27_Modello_SITL_AENEA_2020b/AENEA /AENEA II_SITL1/Forze aerodinamiche/Momenti //press din/Subsystem5 ==
  note: Cn=Cn(alpha_x,beta)+Cn_p*p+Cn_r*r+Cn_deltaA*deltaA+Cn_deltaR*deltaR
  Vect_Costanti : Inport
  Vect_Comandi : Inport  Port=2
  "Vbpolare " : Inport  Port=3
  ωb : Inport  Port=4
  2-D Lookup Table : Lookup_n-D  BreakpointsForDimension1=alphavec_rad  BreakpointsForDimension2=betavec_rad  Table=Cn(2:end,2:end)  InternalRulePriority=Speed  RndMeth=Simplest  InputSameDT=on
      settings: InputPortMap=u0,u1
  Bus Selector : BusSelector  OutputSignals=deltaA,deltaR
  Bus Selector1 : BusSelector  OutputSignals=Coef_Aerodinamici.Coef_Momenti.Cnr,Coef_Geometrici.b/2,Coef_Aerodinamici.Coef_Momenti.Cnp,Coef_Aerodinamici.Coef_Momenti.CndA,Coef_Aerodinamici.Coef_Momenti.CndR
  Bus Selector2 : BusSelector  OutputSignals=α,β,V
  Bus Selector3 : BusSelector  OutputSignals=p,q,r
  Mux : Mux
  Mux1 : Mux
  Product2 : Product
  Product3 : Product
  Sum : Sum  Inputs=5
  Terminator : Terminator
  "controllo divisione per zero np " : MATLAB Function  TreatAsAtomicUnit=on
  "controllo divisione per zero nr " : MATLAB Function  TreatAsAtomicUnit=on
  Cn : Outport  VectorParamsAs1DForOutWhenUnconnected=off
  wires:
  Bus Selector1/3 -> Mux1/1  "<Cnp>"
  Product2/1 -> Sum/4
  Product3/1 -> Sum/5
  Sum/1 -> Cn/1
  Bus Selector1/1 -> Mux/1  "<Cnr>"
  Bus Selector1/5 -> Product3/1  "<CndR>"
  Bus Selector/2 -> Product3/2  "<deltaR>"
  Bus Selector/1 -> Product2/2  "<deltaA>"
  2-D Lookup Table/1 -> Sum/1
  Vect_Comandi/1 -> Bus Selector/1
  Vect_Costanti/1 -> Bus Selector1/1
  Bus Selector1/4 -> Product2/1  "<CndA>"
  Bus Selector1/2 -> Mux1/3, Mux/3  "<b/2>"
  Bus Selector2/3 -> Mux1/4, Mux/4  "<V>"
  "Vbpolare "/1 -> Bus Selector2/1
  Bus Selector2/1 -> 2-D Lookup Table/1  "<α>"
  Bus Selector2/2 -> 2-D Lookup Table/2  "<β>"
  ωb/1 -> Bus Selector3/1
  Bus Selector3/3 -> Mux/2  "<r>"
  Bus Selector3/1 -> Mux1/2  "<p>"
  Bus Selector3/2 -> Terminator/1  "<q>"
  Mux/1 -> "controllo divisione per zero nr "/1(u)
  "controllo divisione per zero nr "/1(y) -> Sum/3
  Mux1/1 -> "controllo divisione per zero np "/1(u)
  "controllo divisione per zero np "/1(y) -> Sum/2

== matlab function v2021_10_27_Modello_SITL_AENEA_2020b/ 1/GPS1/Subsystem2/0-2pi Wrapper ==
  data: a input; y output
function y = fcn(a)
%% Wrapper da [-180,+180] a [0,360]
%https://stackoverflow.com/questions/11498169/dealing-with-angle-wrap-in-c-code
close all

b=2*pi;

k=floor(a/b);
fmod=a-k*b;


if fmod<0
    
   fmod=fmod+2*pi;
    
end

y=fmod;

== stateflow chart v2021_10_27_Modello_SITL_AENEA_2020b/INTERRUTTORI /Chart4  ==
  state manuale
    during:
    man=1;
  state automatico
    during:
    man=1;
  (default) -> manuale
  manuale -> automatico : [t==300]
  data: t input; man output double

== matlab function v2021_10_27_Modello_SITL_AENEA_2020b/AENEA /toSensors/MATLAB Function ==
  data: u input; y output
function y = fcn(u)
omega=[u(1),u(2),u(3)];
rAHRSG=[u(4),u(5),u(6)];

if length(omega)==3 & length(rAHRSG)==3
    y1=cross(omega,rAHRSG);
    y=cross(omega,y1);
else 
    error('input diension incorrect')
end

== matlab function v2021_10_27_Modello_SITL_AENEA_2020b/AENEA /AENEA II_SITL1/Forze aerodinamiche/Forze assi vento//q/Subsystem1/controllo divisione per zero Yp  ==
  data: u input; y output
function y = Yp(u)

if length(u)~=4
    error('vettore ingresso dimensione errata')
else
    if u(4)==0
        y=0;
    else
        y=u(1)*u(2)*u(3)/u(4);
    end
end

== matlab function v2021_10_27_Modello_SITL_AENEA_2020b/AENEA /AENEA II_SITL1/Forze aerodinamiche/Forze assi vento//q/Subsystem1/controllo divisione per zero Yr ==
  data: u input; y output
function y = Yr(u)

if length(u)~=4
    error('vettore ingresso dimensione errata')
else
    if u(4)==0
        y=0;
    else
        y=u(1)*u(2)*u(3)/u(4);
    end
end

== matlab function v2021_10_27_Modello_SITL_AENEA_2020b/AENEA /AENEA II_SITL1/Forze aerodinamiche/Forze assi vento//q/Subsystem2/controllo divisione per zero Lq  ==
  data: u input; y output
function y = Lq(u)

if length(u)~=4
    error('vettore ingresso dimensione errata')
else
    if u(4)==0
        y=0;
    else
        y=u(1)*u(2)*u(3)/u(4);
    end
end

== matlab function v2021_10_27_Modello_SITL_AENEA_2020b/AENEA /AENEA II_SITL1/Forze aerodinamiche/MATLAB Function ==
  data: alpha input; Lbw output; beta input
function Lbw = DCMbw(alpha,beta)


Lbw=[cos(alpha)*cos(beta), -cos(alpha)*sin(beta), -sin(alpha); sin(beta), cos(beta), 0; sin(alpha)*cos(beta), -sin(alpha)*sin(beta), cos(alpha)];

== matlab function v2021_10_27_Modello_SITL_AENEA_2020b/AENEA /AENEA II_SITL1/Forze aerodinamiche/Momenti //press din/Subsystem3/controllo divisione per zero lp  ==
  data: u input; y output
function y = lp(u)

if length(u)~=4
    error('vettore ingresso dimensione errata')
else
    if u(4)==0
        y=0;
    else
        y=u(1)*u(2)*u(3)/u(4);
    end
end

== matlab function v2021_10_27_Modello_SITL_AENEA_2020b/AENEA /AENEA II_SITL1/Forze aerodinamiche/Momenti //press din/Subsystem3/controllo divisione per zero lr  ==
  data: u input; y output
function y = lr(u)

if length(u)~=4
    error('vettore ingresso dimensione errata')
else
    if u(4)==0
        y=0;
    else
        y=u(1)*u(2)*u(3)/u(4);
    end
end

== matlab function v2021_10_27_Modello_SITL_AENEA_2020b/AENEA /AENEA II_SITL1/Forze aerodinamiche/Momenti //press din/Subsystem4/controllo divisione per zero mq  ==
  data: u input; y output
function y = mq(u)

if length(u)~=4
    error('vettore ingresso dimensione errata')
else
    if u(4)==0
        y=0;
    else
        y=u(1)*u(2)*u(3)/u(4);
    end
end

== matlab function v2021_10_27_Modello_SITL_AENEA_2020b/AENEA /AENEA II_SITL1/Forze aerodinamiche/Momenti //press din/Subsystem5/controllo divisione per zero np  ==
  data: u input; y output
function y = np(u)

if length(u)~=4
    error('vettore ingresso dimensione errata')
else
    if u(4)==0
        y=0;
    else
        y=u(1)*u(2)*u(3)/u(4);
    end
end

== stateflow chart v2021_10_27_Modello_SITL_AENEA_2020b/INTERRUTTORI /Chart5 ==
  state GC_info1
    during:
    GC_info=1;
  state GC_info
    during:
    GC_info=1;
  state GC_info2
    during:
    GC_info=1;
  (default) -> GC_info
  GC_info -> GC_info1 : [t==60]
  GC_info1 -> GC_info2 : [t==61]
  data: t input; GC_info output double

== matlab function v2021_10_27_Modello_SITL_AENEA_2020b/AENEA /AENEA II_SITL1/Forze aerodinamiche/Momenti //press din/Subsystem5/controllo divisione per zero nr  ==
  data: u input; y output
function y = nr(u)

if length(u)~=4
    error('vettore ingresso dimensione errata')
else
    if u(4)==0
        y=0;
    else
        y=u(1)*u(2)*u(3)/u(4);
    end
end

== matlab function v2021_10_27_Modello_SITL_AENEA_2020b/AENEA /AENEA II_SITL1/MATLAB Function ==
  data: PHI input; invR output
function invR = omega2PHIdot(PHI)

if length(PHI)==3
    Phi=PHI(1);
    Theta=PHI(2);
    
    invR=[1, sin(Phi)*tan(Theta), cos(Phi)*tan(Theta); 0, cos(Phi), -sin(Phi); 0, sin(Phi)*sec(Theta), cos(Phi)*sec(Theta)];
else 
    error('il vettore PHI non va bene')
end

== matlab function v2021_10_27_Modello_SITL_AENEA_2020b/AENEA /AENEA II_SITL1/Propulsione1/LUT ELICA /MATLAB Function ==
  data: J input; Ct output; RPM input; Cp output; matricepolinomi input
function [Ct,Cp] = calcolo_Ct_Cp(J,RPM,matricepolinomi)

lct00 = matricepolinomi(1,1);
lct10 = matricepolinomi(1,2);
lct01 = matricepolinomi(1,3);
lct20 = matricepolinomi(1,4);
lct11 = matricepolinomi(1,5);
lct02 = matricepolinomi(1,6);
lct30 = matricepolinomi(1,7);
lct21 = matricepolinomi(1,8);
lct12 = matricepolinomi(1,9);
lct40 = matricepolinomi(1,10);
lct31 = matricepolinomi(1,11);
lct22 = matricepolinomi(1,12);

qct00 = matricepolinomi(2,1);
qct10 = matricepolinomi(2,2);
qct01 = matricepolinomi(2,3);
qct20 = matricepolinomi(2,4);
qct11 = matricepolinomi(2,5);
qct02 = matricepolinomi(2,6);
qct30 = matricepolinomi(2,7);
qct21 = matricepolinomi(2,8);
qct12 = matricepolinomi(2,9);
qct03 = matricepolinomi(2,10);
qct40 = matricepolinomi(2,11);
qct31 = matricepolinomi(2,12);
qct22 = matricepolinomi(2,13);
qct13 = matricepolinomi(2,14);
qct04 = matricepolinomi(2,15);
qct50 = matricepolinomi(2,16);
qct41 = matricepolinomi(2,17);
qct32 = matricepolinomi(2,18);
qct23 = matricepolinomi(2,19);
qct14 = matricepolinomi(2,20);
qct05 = matricepolinomi(2,21);

cp100 = matricepolinomi(3,1);
cp110 = matricepolinomi(3,2);
cp101 = matricepolinomi(3,3);
cp120 = matricepolinomi(3,4);
cp111 = matricepolinomi(3,5);
cp102 = matricepolinomi(3,6);
cp130 = matricepolinomi(3,7);
cp121 = matricepolinomi(3,8);
cp112 = matricepolinomi(3,9);
cp140 = matricepolinomi(3,10);
cp131 = matricepolinomi(3,11);
cp122 = matricepolinomi(3,12);

cp200 = matricepolinomi(4,1);
cp210 = matricepolinomi(4,2);
cp201 = matricepolinomi(4,3);
cp220 = matricepolinomi(4,4);
cp211 = matricepolinomi(4,5);
cp202 = matricepolinomi(4,6);
cp230 = matricepolinomi(4,7);
cp221 = matricepolinomi(4,8);
cp212 = matricepolinomi(4,9);
cp240 = matricepolinomi(4,10);
cp231 = matricepolinomi(4,11);
cp222 = matricepolinomi(4,12);

cp300 = matricepolinomi(5,1);
cp310 = matricepolinomi(5,2);
cp301 = matricepolinomi(5,3);
cp320 = matricepolinomi(5,4);
cp311 = matricepolinomi(5,5);
cp302 = matricepolinomi(5,6);
cp330 = matricepolinomi(5,7);
cp321 = matricepolinomi(5,8);
cp312 = matricepolinomi(5,9);
cp340 = matricepolinomi(5,10);
cp331 = matricepolinomi(5,11);
cp322 = matricepolinomi(5,12);

cp400 = matricepolinomi(6,1);
cp410 = matricepolinomi(6,2);
cp401 = matricepolinomi(6,3);
cp420 = matricepolinomi(6,4);
cp411 = matricepolinomi(6,5);
cp402 = matricepolinomi(6,6);
cp430 = matricepolinomi(6,7);
cp421 = matricepolinomi(6,8);
cp412 = matricepolinomi(6,9);
cp440 = matricepolinomi(6,10);
cp431 = matricepolinomi(6,11);
cp422 = matricepolinomi(6,12);


if J<=0.32
    x = RPM;
    y = J;
    Ct = qct00 + qct10*x + qct01*y + qct20*x^2 + qct11*x*y + qct02*y^2 + qct30*x^3 + qct21*x^2*y + qct12*x*y^2 + qct03*y^3 + qct40*x^4 + qct31*x^3*y + qct22*x^2*y^2 + qct13*x*y^3 + qct04*y^4 + qct50*x^5 + qct41*x^4*y + qct32*x^3*y^2 + qct23*x^2*y^3 + qct14*x*y^4 + qct05*y^5;
elseif J>0.32
    x = RPM;
    y = J;
    Ct = lct00 + lct10*x + lct01*y + lct20*x^2 + lct11*x*y + lct02*y^2 + lct30*x^3 + lct21*x^2*y + lct12*x*y^2 + lct40*x^4 + lct31*x^3*y + lct22*x^2*y^2;
else
    Ct = 0;
end

if (J<=0.34)&&(RPM<=5000)
    x = RPM;
    y = J;
    Cp = cp100 + cp110*x + cp101*y + cp120*x^2 + cp111*x*y + cp102*y^2 + cp130*x^3 + cp121*x^2*y + cp112*x*y^2 + cp140*x^4 + cp131*x^3*y + cp122*x^2*y^2;
elseif (J<=0.34)&&(RPM>5000)
    x = RPM;
    y = J;
    Cp = cp200 + cp210*x + cp201*y + cp220*x^2 + cp211*x*y + cp202*y^2 + cp230*x^3 + cp221*x^2*y + cp212*x*y^2 + cp240*x^4 + cp231*x^3*y + cp222*x^2*y^2;
elseif (J>0.34)&&(RPM<=5000)
    x = RPM;
    y = J;
    Cp = cp300 + cp310*x + cp301*y + cp320*x^2 + cp311*x*y + cp302*y^2 + cp330*x^3 + cp321*x^2*y + cp312*x*y^2 + cp340*x^4 + cp331*x^3*y + cp322*x^2*y^2;
elseif (J>0.34)&&(RPM>5000)
    x = RPM;
    y = J;
    Cp = cp400 + cp410*x + cp401*y + cp420*x^2 + cp411*x*y + cp402*y^2 + cp430*x^3 + cp421*x^2*y + cp412*x*y^2 + cp440*x^4 + cp431*x^3*y + cp422*x^2*y^2;
else
    Cp = 0;
end

== matlab function v2021_10_27_Modello_SITL_AENEA_2020b/AENEA /AENEA II_SITL1/Velocità1/MATLAB Function ==
  data: V input; module output
function module = absolute(V)

module=sqrt((V(1)^2)+(V(2)^2)+(V(3)^2));

end

== matlab function v2021_10_27_Modello_SITL_AENEA_2020b/AENEA /AENEA II_SITL1/Velocità1/controllo divisione per 0 su alpha ==
  data: u input; y output
function y = tgalpha(u)

if length(u)~=2
    error('vettore ingresso errato')
else
    if u(2)==0
        y=0;
    else 
        y=u(1)/u(2);
    end
end

== matlab function v2021_10_27_Modello_SITL_AENEA_2020b/AENEA /AENEA II_SITL1/Velocità1/controllo divisione per 0 su beta ==
  data: u input; y output
function y = sinbeta(u)

if length(u)~=2
    error('vettore ingresso errato')
else
    if u(2)==0
        y=0;
    else 
        y=u(1)/u(2);
    end
end

== stateflow chart v2021_10_27_Modello_SITL_AENEA_2020b/RIFERIMENTI/Chart3 ==
  state manuale
    during:
    VEL=20;
  state automatico
    during:
    VEL=17;
  (default) -> manuale
  manuale -> automatico : [t==100]
  data: t input; ROTTA output double

== stateflow chart v2021_10_27_Modello_SITL_AENEA_2020b/INTERRUTTORI /Chart2 ==
  state ALsi
    during:
    AL=1;
  state ALno
    during:
    AL=0;
  (default) -> ALno
  ALno -> ALsi : [t==30]
  data: t input; AL output double

== matlab function v2021_10_27_Modello_SITL_AENEA_2020b/AENEA /AENEA II_SITL1/Velocità1/MATLAB Function1 ==
  data: V input; module output
function module = absolute(V)

module=sqrt((V(1)^2)+(V(2)^2)+(V(3)^2));

end

== stateflow chart v2021_10_27_Modello_SITL_AENEA_2020b/INTERRUTTORI /Chart1 ==
  state automatico
    during:
    man=0;
  state manuale
    during:
    man=1;
  (default) -> manuale
  manuale -> automatico : [t==5]
  data: t input; man output double

== matlab function v2021_10_27_Modello_SITL_AENEA_2020b/ 1/BMP 280/MATLAB Function1 ==
  data: h input; P_ output; T0ref input; P_ref input
function P_ = pbaro_rev(h,T0ref,P_ref)


g     = 9.81;    %accelerazione di gravità
R_gas = 287.05;  %costante dei gas perfetti
dTdh  = -0.0065; %gradiente termico verticale in atmosfera standard 

T_0 = T0ref+273.15;

% P_ref = 1.0074e+05;

% a=h/((((R_gas*T_0)/g)+dTdh*0.5*R_gas/g*h));

a=h/(((R_gas*T_0)/g)+h*dTdh*0.5*(R_gas/g));

P_=P_ref/exp(a);
end

== matlab function v2021_10_27_Modello_SITL_AENEA_2020b/ 1/BMP 280/MATLAB Function3 ==
  data: P input; h_ output; T0ref input; P_ref input
function h_ = hbaro(P,T0ref,P_ref)


g     = 9.81;    %accelerazione di gravità
R_gas = 287.05;  %costante dei gas perfetti
dTdh  = -0.0065; %gradiente termico verticale in atmosfera standard 

T_0 = T0ref+273.15;


% P_ref = 1.0073e+05;
    
h_ = ((R_gas/g)*log(P_ref/P)*T_0)/(1-(dTdh*0.5*(R_gas/g)*log(P_ref/P)));
end

== matlab function v2021_10_27_Modello_SITL_AENEA_2020b/ 1/Correzione PSI ==
  data: psi input; y output; psi_k input
function y  = fcn(psi,psi_k)
%% Correzione ingresso psi
persistent salto

if isempty(salto)
    salto=0;
end


  if psi_k<0 && psi>0 && psi-psi_k > pi/2
      
       salto = salto-2*pi;
     
  end
  
  if psi_k>0 && psi<0 && psi_k-psi > pi/2
      
       salto = salto+2*pi;

  end
  
  y= (psi+salto);


%   salto_out=salto;

end
%%

== stateflow chart v2021_10_27_Modello_SITL_AENEA_2020b/RIFERIMENTI/Chart1 ==
  state manuale
    during:
    QUOTA=100;
  state automatico
    during:
    QUOTA=200;
  state automatico1
    during:
    QUOTA=50;
  (default) -> manuale
  automatico -> automatico1 : [t==200]
  manuale -> automatico : [t==100]
  data: t input; QUOTA output double

== stateflow chart v2021_10_27_Modello_SITL_AENEA_2020b/RIFERIMENTI/Chart2 ==
  state manuale
    during:
    ROTTA=0;
  state automatico
    during:
    ROTTA=45;
  (default) -> manuale
  manuale -> automatico : [t==60]
  data: t input; ROTTA output double
